simulink model "Bilateral_Ankle_Exo"  (R2017b)
settings: Solver=ode1  StartTime=0.0  StopTime=Inf  FixedStep=0.0002  RelTol=1e-3
PostLoadFcn:
  | , if any(exist('dsrtsu_mdlpostloadfcn', 'file') == [2, 3, 6]), try dsrtsu_mdlpostloadfcn('Execute', bdroot); catch fprintf('Error in PostLoadFcn (dsrtsu_mdlpostloadfcn) for model "%s":\n %s\n', bdroot, lasterr); end, end,
libraries: dsparch4 x12, rti1202lib_dio_class1 x8, rti1202lib_adc_class1 x8, rtican x5, rtiemclib x4, rti1202lib_dac_class1 x2, dsextras x1, rti1202lib_base x1, rtitasklib x1
(part 4 of 4)

== system Bilateral_Ankle_Exo/Sensor Data/IMU module/IMU/Subsystem6 ==
  Accel : Inport
  Data Type Conversion : DataTypeConversion  OutDataTypeStr=double
  Gain : Gain  Gain=4/32767
  Out1 : Outport
  wires:
  Data Type Conversion/1 -> Gain/1
  Gain/1 -> Out1/1
  Accel/1 -> Data Type Conversion/1

== system Bilateral_Ankle_Exo/Sensor Data/IMU module/IMU/Subsystem7 ==
  Accel : Inport
  Data Type Conversion : DataTypeConversion  OutDataTypeStr=double
  Gain : Gain  Gain=4/32767
  Out1 : Outport
  wires:
  Data Type Conversion/1 -> Gain/1
  Gain/1 -> Out1/1
  Accel/1 -> Data Type Conversion/1

== system Bilateral_Ankle_Exo/Sensor Data/IMU module/IMU/Subsystem8 ==
  Accel : Inport
  Data Type Conversion : DataTypeConversion  OutDataTypeStr=double
  Gain : Gain  Gain=4/32767
  Out1 : Outport
  wires:
  Data Type Conversion/1 -> Gain/1
  Gain/1 -> Out1/1
  Accel/1 -> Data Type Conversion/1

== system Bilateral_Ankle_Exo/RTI Data/RTI Data Store/RTI Data Store/RTI Data Store/RTI Data Store ==

== matlab function Bilateral_Ankle_Exo/Sensor Data/Ankle Encoder/Calibration_R ==
  data: encoder input; angle output; BT_RESET_ANKLE_R parameter boolean; ParmReg_R data_store_memory
function angle = process(encoder, BT_RESET_ANKLE_R)
    global ParmReg_R;
    angle_zero = ParmReg_R(3);


    if BT_RESET_ANKLE_R == 1
        angle_zero = encoder;
        ParmReg_R(3) = angle_zero;
    end

    angle = encoder - angle_zero;
end

== matlab function Bilateral_Ankle_Exo/Sensor Data/Motor Encoder/Calibration_L ==
  data: encoder input; BT_RESET_MOTOR_L parameter boolean; angle output; ParmReg_L data_store_memory
function angle = process(encoder, BT_RESET_MOTOR_L)
    global ParmReg_L;
    angle_zero = ParmReg_L(2);

    if BT_RESET_MOTOR_L == 1
        angle_zero = encoder;
        ParmReg_L(2) = angle_zero;
    end

    angle = encoder - angle_zero;
    
end

== matlab function Bilateral_Ankle_Exo/Sensor Data/Ankle Encoder/Mux ==
  data: x1 input; x output; x2 input
function x = mux(x1,x2)

x = [x1 x2];

== matlab function Bilateral_Ankle_Exo/Sensor Data/Torque module/Calibration_R ==
  data: vol input; torque output; load_vol_gain parameter double; load_vol_offset parameter double; BT_RESET_TORQUE_R parameter boolean; ParmReg_R data_store_memory
function torque = process(vol, load_vol_gain, load_vol_offset, BT_RESET_TORQUE_R)
%% 功能：电压-力矩转换与力矩归零
    global ParmReg_R;
    torque_zero = ParmReg_R(1);

    %%% 力矩归零
    if BT_RESET_TORQUE_R == 1
        torque_zero = vol*load_vol_gain + load_vol_offset;
        ParmReg_R(1) = torque_zero;
    end

    torque = vol*load_vol_gain + load_vol_offset - torque_zero;

end

== matlab function Bilateral_Ankle_Exo/Sensor Data/Motor Encoder/Mux1 ==
  data: x1 input; x output; x2 input; x3 input
function x = mux(x1,x2,x3)

x = [x1 x2 x3];

== matlab function Bilateral_Ankle_Exo/Sensor Data/FootSwitch module/Filter_R ==
  data: signal input; state output
function state = filter(signal)

%% 对足底开关信号进行滤波
% 滤波原则：上升沿无滤波，下降沿消抖滤波

Ts = 0.0002;
persistent foot_state;
persistent filter_time;

if isempty(foot_state)
    foot_state = 0;
    filter_time = 0;
end

if foot_state == 0
    if signal == 1
        foot_state = 1;
    else
        foot_state = 0;
    end
else
    if signal == 1
        foot_state = 1;
    else
        filter_time = filter_time + Ts;
        if filter_time > 0.1
            filter_time = 0;
            foot_state = 0;
        end
    end
end

state = foot_state;

end

== matlab function Bilateral_Ankle_Exo/Parameter Module/Control Parameter/Mux1 ==
  data: x1 input; x output; x2 input; x3 input; x4 input; x5 input; x6 input; reset input
function x = mux(x1,x2,x3,x4,x5,x6, reset)

if reset == 1
    x = [0 0 0 0 0 0];
else
    x = [x1 x2 x3 x4 x5 x6];
end

== matlab function Bilateral_Ankle_Exo/Parameter Module/Torque Parameter/Mux1 ==
  data: x1 input; x output; x2 input; x3 input; x4 input
function x = mux(x1,x2,x3,x4)

x = [x1 x2 x3,x4];

== matlab function Bilateral_Ankle_Exo/State_Module_r/State Machine ==
  data: mode_r output; footswitch_r input; state_r output; BT_RUN_R parameter boolean; BT_SLACK_R parameter boolean; BT_IDLE_R parameter boolean; BT_ERROR_R parameter boolean; stride_time_r output; BT_CALIB_R parameter boolean; stride_timer_r output
function [mode_r,state_r,stride_time_r,stride_timer_r] = StateMechine(footswitch_r, BT_RUN_R, BT_SLACK_R, BT_IDLE_R, BT_ERROR_R, BT_CALIB_R)

%% 定义寄存变量
persistent reg_stride_time;
persistent reg_stride_time_count;
persistent reg_mode;
persistent reg_state;
persistent bt_run;
persistent reg_last_switch;

if isempty(reg_stride_time)
    reg_stride_time = 1;
    reg_stride_time_count = 0;
    reg_mode = 1;
    reg_state = 1;
    bt_run = 0;
    reg_last_switch = 1;
end

%% 参数定义
Ts = 0.0002;
PP_StandSwing = 0.65;
max_stride_time = 1.5;
min_sride_time = 0.5;

%% 模式说明
IDLE_MODE  = 1;
WALK_MODE   = 2;
SLACK_MODE = 3;
CALIB_MODE = 4;
ERROR_MODE = 0;

%% 模式转换
if BT_RUN_R == 1
    bt_run = 1;
end
if BT_CALIB_R == 1
    reg_mode = CALIB_MODE;
end
if BT_SLACK_R == 1
    reg_mode = SLACK_MODE;
end
if BT_IDLE_R == 1
    reg_mode = IDLE_MODE;
end
if BT_ERROR_R == 1
    reg_mode = ERROR_MODE;
end
% 运行模式在swing->stance时切换
if bt_run == 1 && reg_last_switch == 0 && footswitch_r == 1
    reg_mode = WALK_MODE;
    bt_run = 0;
end
        
if reg_mode == WALK_MODE || reg_mode == IDLE_MODE
    if reg_last_switch == 0 && footswitch_r == 1
        reg_state = 1;
        
        if reg_stride_time_count < max_stride_time && reg_stride_time_count > min_sride_time
            reg_stride_time = 0.618*reg_stride_time + 0.382*reg_stride_time_count;
        end
        
        reg_stride_time_count = 0;
        
    elseif reg_state ==1 && reg_stride_time_count > PP_StandSwing * reg_stride_time
        reg_state = 0;
        reg_stride_time_count = reg_stride_time_count + Ts;
    else
        reg_stride_time_count = reg_stride_time_count + Ts;
    end
end

reg_last_switch = footswitch_r;
if reg_stride_time > max_stride_time
    reg_stride_time = max_stride_time;
elseif reg_stride_time < min_sride_time
    reg_stride_time = min_sride_time;
end

mode_r = reg_mode;
state_r = reg_state;
stride_time_r = reg_stride_time;
stride_timer_r = reg_stride_time_count;

end

== matlab function Bilateral_Ankle_Exo/State_Module_r/Mux1 ==
  data: x1 input; x output; x2 input; x3 input; x4 input
function x = mux(x1,x2,x3,x4)

x = [x1 x2 x3,x4];

== matlab function Bilateral_Ankle_Exo/Control Module/Controller_R ==
  data: state input; motor_vel_cmd_r output; torque input; ankle input; motor input; control_parm input; torque_trace_des input; torque_delta_trace_des input; lrn_cmd input; MODE_R parameter int8; FOLLOW_SLACK_ANGLE_R parameter double; TorqueMem_R data_store_memory; SWING_MAX_ANGLE_R parameter double; ParmReg_R data_store_memory
function motor_vel_cmd_r  = control(state,torque,ankle,motor,control_parm,torque_trace_des,torque_delta_trace_des,lrn_cmd, MODE_R,FOLLOW_SLACK_ANGLE_R,SWING_MAX_ANGLE_R)

global ParmReg_R;

%% 寄存变量声明
persistent calib_state;
persistent smooth_filter;
if isempty(calib_state)
    calib_state = 0;
    smooth_filter = 0;
end

%% 模式定义
IDLE_MODE  = 1;
WALK_MODE   = 2;
SLACK_MODE = 3;
CALIB_MODE = 4;
ERROR_MODE = 0;

%% 控制模式定义
FOLLOW_MODE = 1;
TORQUE_MODE = 2;

%% 参数定义
GearRatio = 5;
RadiusRatio = 40/108;
MotorTimeConstance = 0.05;
CALIB_SPEED = 30;
SLACK_SPEED = 30;
CALIB_TORQUE = 5;
CALIB_SLACK_ANGLE = 20;

%% 数据提取
STATE = state(1);
footstate = state(2);
stride_time = state(3);
stride_timer = state(4);

ankle_angle = ankle(1);
ankle_gyro = ankle(2);
motor_angle = motor(1);
motor_gyro = motor(2);

torque_measure = torque(1);
torque_delta = torque(2);
torque_des = torque_trace_des;
torque_delta_des = torque_delta_trace_des;

Kp = control_parm(1);
Kd = control_parm(2);
Ksp = control_parm(4);
Ksd = control_parm(5);
Ko = control_parm(6);
Ks = 2;

switch STATE
    case IDLE_MODE
        motor_vel_cmd_r = 0;
        calib_state = 0;
        
    case SLACK_MODE
        motor_vel_cmd_r = -SLACK_SPEED*GearRatio;
        
    case CALIB_MODE
        if calib_state == 0 && torque_measure < CALIB_TORQUE
            motor_vel_cmd_r = CALIB_SPEED*GearRatio;
        elseif calib_state == 0 && torque_measure > CALIB_TORQUE
            calib_state = 1;
            motor_vel_cmd_r = 0;
            motor_angle_zero = ParmReg_R(2) + motor_angle - CALIB_SLACK_ANGLE;
            ParmReg_R(2) = motor_angle_zero;
        else
            motor_vel_cmd_r = 0;
        end
        
    case WALK_MODE
        switch MODE_R
            
            case FOLLOW_MODE
                angle_error = ankle_angle - FOLLOW_SLACK_ANGLE_R - motor_angle*RadiusRatio;
                gyro_error = ankle_gyro*RadiusRatio;
                motor_vel_cmd_r = (Ksp*angle_error  + Ksd*gyro_error)*GearRatio/MotorTimeConstance;
                
            case TORQUE_MODE
                if footstate == 1
                    torque_error = torque_des - torque_measure;
                    torque_delta_error = torque_delta_des - torque_delta;
                    speed_des = Ko*torque_delta_des;
                    
                    angle_error = ankle_angle - FOLLOW_SLACK_ANGLE_R - motor_angle*RadiusRatio;
                    gyro_error = ankle_gyro*RadiusRatio;
                    motor_vel_cmd_r = (Ksp*angle_error  + Ksd*gyro_error)*GearRatio/MotorTimeConstance;
                    
                    if torque_des < 0.001
                        smooth_filter = smooth_filter + 0.05;
                        if smooth_filter > 1
                            smooth_filter = 1;
                        end
                    else
                        smooth_filter = 0;
                    end
                    
                    motor_vel_cmd_r = ((1-smooth_filter)*(Kp*torque_error + Kd*torque_delta_error + lrn_cmd + speed_des) + smooth_filter*(Ksp*angle_error  + Ksd*gyro_error)) * GearRatio / MotorTimeConstance;
                else
%                     angle_error = 0 - motor_angle*RadiusRatio;
%                     motor_vel_cmd = ( Ks * angle_error ) * GearRatio / MotorTimeConstance;
                    smooth_filter = 0;
                    angle_error = ankle_angle - FOLLOW_SLACK_ANGLE_R - motor_angle*RadiusRatio;
                    gyro_error = ankle_gyro*RadiusRatio;
                    motor_vel_cmd_r = (Ksp*angle_error  + Ksd*gyro_error)*GearRatio/MotorTimeConstance;
                end
            otherwise
                motor_vel_cmd_r = 0;
        end
        
    case ERROR_MODE
        motor_vel_cmd_r = 0;
        
    otherwise
        motor_vel_cmd_r = 0;
end


end

== matlab function Bilateral_Ankle_Exo/Control Module/Motor_R/MATLAB Function ==
  data: torque input; vel output; ankle input; motor input; motor_vel_cmd input; MAX_TORQUE parameter double; MAX_MOTOR_ANGLE parameter double; MIN_MOTOR_ANGLE parameter double; MAX_SPEED parameter double
function vel = fcn(torque,ankle,motor,motor_vel_cmd,MAX_TORQUE, MAX_MOTOR_ANGLE, MIN_MOTOR_ANGLE, MAX_SPEED)

motor_angle = motor(1);
torque_measure = torque(1);

if torque_measure > MAX_TORQUE
    vel = 0;
elseif motor_angle > MAX_MOTOR_ANGLE
    vel = 0;
elseif motor_angle < MIN_MOTOR_ANGLE
    vel = 0;
elseif motor_vel_cmd > MAX_SPEED
    vel = MAX_SPEED;
elseif motor_vel_cmd < - MAX_SPEED
    vel = - MAX_SPEED;
else
    vel = motor_vel_cmd;
end

end

== matlab function Bilateral_Ankle_Exo/Control Module/Torque Track R ==
  data: torque_parm_r input; torque_r input; torque_des_r output; torque_delta_des_r output; state_r input; TorqueMem_R data_store_memory; torque_trace_r output; torque_delta_trace_r output; torque_offset_r input; torque_error_r output
function [torque_des_r,torque_delta_des_r,torque_trace_r,torque_delta_trace_r,torque_error_r] = TorqueTrack(torque_parm_r,torque_r,state_r, torque_offset_r)

%% 寄存变量声明
global TorqueMem_R;

persistent last_footstate;
if isempty(last_footstate)
    last_footstate = 0;
end

%% 参数定义
Fs = 500;

%% 模式定义
IDLE_MODE  = 1;
WALK_MODE   = 2;

%% 数据提取
mode = state_r(1);
footstate = state_r(2);
stride_time = state_r(3);
stride_timer = state_r(4);

peak_torque = torque_parm_r(1);
rise_time = torque_parm_r(2);
peak_time = torque_parm_r(3);
fall_time = torque_parm_r(4);

torque_measure = torque_r(1);
troque_delta = torque_r(2);
stride_index = stride_timer*Fs + 1;
if stride_index > 750
    stride_index = 750;
end

%% 更新期望力矩曲线
if last_footstate == 0 && footstate == 1 && (mode == WALK_MODE || mode == IDLE_MODE)
    
    torque_track = zeros(1,750);
    
    torque_delta_track = zeros(1,750);
    time_index = 1:750;
    one_line = ones(1,750);
    index_peak = floor(peak_time/100*stride_time*Fs);
    index_rise = index_peak - floor(rise_time/100*stride_time*Fs);
    index_fall = index_peak + floor(fall_time/100*stride_time*Fs);
    
    %rise time前预拉紧阶段  ->使用向量代替循环以提高效率
    torque_track(1:floor(index_rise-1)) = time_index(1:floor(index_rise-1))/index_rise * torque_offset_r;
    
    % 上升阶段
    % 构造三次样条函数方程组
    A1 = [1,index_rise,index_rise^2,index_rise^3;
          1,index_peak,index_peak^2,index_peak^3;
          0,1,2*index_rise,3*index_rise^2;
          0,1,2*index_peak,3*index_peak^2];
    b1 = [torque_offset_r;peak_torque;0;0];
    parm1 = (A1\b1)';
    torque_track(floor(index_rise):floor(index_peak-1)) = parm1*[one_line(1:floor(index_peak-index_rise));time_index(floor(index_rise):floor(index_peak-1));time_index(floor(index_rise):floor(index_peak-1)).^2;time_index(floor(index_rise):floor(index_peak-1)).^3];
    torque_delta_track(index_rise:index_peak-1) = parm1(2:4)*[one_line(1:index_peak-index_rise);2*time_index(index_rise:index_peak-1);3*time_index(index_rise:index_peak-1).^2]*Fs;
    
    % 下降阶段
    A2 = [1,index_peak,index_peak^2,index_peak^3;
          1,index_fall,index_fall^2,index_fall^3;
          0,1,2*index_peak,3*index_peak^2;
          0,1,2*index_fall,3*index_fall^2];
    b2 = [peak_torque;0;0;0];
    parm2 = (A2\b2)';
    torque_track(floor(index_peak):floor(index_fall)) = parm2*[one_line(1:floor(index_fall+1-index_peak));time_index(floor(index_peak):floor(index_fall));time_index(floor(index_peak):floor(index_fall)).^2;time_index(floor(index_peak):floor(index_fall)).^3];
    
    %--------------------
    TorqueMem_R(1,1:750) = torque_track(1:750);
    %TorqueMem(2,1:750) = zeros(1,750);
    TorqueMem_R(3,1:750) = torque_delta_track(1:750);
    %TorqueMem(4,1:750) = zeros(1,750);
end

last_footstate = footstate;
TorqueMem_R(2,stride_index) = torque_measure;
TorqueMem_R(4,stride_index) = troque_delta;

if mode == WALK_MODE
    torque_des_r = TorqueMem_R(1,stride_index);
    torque_delta_des_r = TorqueMem_R(3,stride_index);
else
    torque_des_r = 0;
    torque_delta_des_r = 0;
end

torque_trace_r = TorqueMem_R(1:2,1:750);
torque_delta_trace_r = TorqueMem_R(3:4,1:750);

torque_error_r = torque_des_r - torque_r;

end

== matlab function Bilateral_Ankle_Exo/Control Module/LRN_R ==
  data: lrn_cmd_r output; state input; control_parm input; torque_parm input; BT_LRN_CLEAR_R parameter boolean; BT_LRN_ON_R parameter boolean; error_filter_k_r parameter double; time_delay_r parameter int32; lrn_mem_r output; TorqueMem_R data_store_memory; lrn_shrink_r parameter double
function [lrn_cmd_r, lrn_mem_r] = LRN_controller(state,control_parm,torque_parm, BT_LRN_CLEAR_R, BT_LRN_ON_R, error_filter_k_r, time_delay_r, lrn_shrink_r)

global TorqueMem_R;

persistent last_footstate;
persistent torque_error_memory;
persistent lrn_cmd_memory;
persistent last_torque_parm;

if isempty(last_footstate)
    last_footstate = 0;
    torque_error_memory = zeros(1,1000);
    lrn_cmd_memory = zeros(1,1000);
    last_torque_parm = [torque_parm(1) torque_parm(3)];
end

%% 参数定义
Fs = 500;

%% 模式定义
IDLE_MODE  = 1;
WALK_MODE   = 2;

%% 数据提取
mode = state(1);
footstate = state(2);
stride_time = state(3);
stride_timer = state(4);

Kl = control_parm(3);

stride_index = stride_timer*Fs + 1;
if stride_index > 750
    stride_index = 750;
end

if last_footstate == 0 && footstate == 1 && mode == WALK_MODE && BT_LRN_ON_R == 1
    error = TorqueMem_R(1,1:750) - TorqueMem_R(2,1:750);
    torque_error_memory(1:750) = (1-error_filter_k_r)*torque_error_memory(1:750) + error_filter_k_r*error;
    lrn_cmd_memory(1:750) = lrn_shrink_r*lrn_cmd_memory(1:750) + Kl*torque_error_memory(1:750);
end
    
if BT_LRN_CLEAR_R == 1 || last_torque_parm(1) ~= torque_parm(1) || last_torque_parm(2) ~= torque_parm(3)
    torque_error_memory = zeros(1,1000);
    lrn_cmd_memory = zeros(1,1000);
end

if mode == WALK_MODE
    if stride_index >= 750 - floor(time_delay_r)
        lrn_cmd_r = 0;
    else
        lrn_cmd_r = lrn_cmd_memory(1,stride_index + floor(time_delay_r));
    end
else
    lrn_cmd_r = 0;
end

last_footstate = footstate;
last_torque_parm = [torque_parm(1) torque_parm(3)];
lrn_mem_r = lrn_cmd_memory(1:750);


end

== matlab function Bilateral_Ankle_Exo/Sensor Data/Torque module/Calibration_L ==
  data: vol input; load_vol_gain parameter double; load_vol_offset parameter double; torque output; ParmReg_L data_store_memory; BT_RESET_TORQUE_L parameter boolean
function torque = process(vol, load_vol_gain, load_vol_offset, BT_RESET_TORQUE_L)
%% 功能：电压-力矩转换与力矩归零
    global ParmReg_L;
    torque_zero = ParmReg_L(1);

    %%% 力矩归零
    if BT_RESET_TORQUE_L == 1
        torque_zero = vol*load_vol_gain + load_vol_offset;
        ParmReg_L(1) = torque_zero;
    end

    torque = vol*load_vol_gain + load_vol_offset - torque_zero;

end

== matlab function Bilateral_Ankle_Exo/Sensor Data/Torque module/Mux_R ==
  data: x1 input; x output; x2 input
function x = mux(x1,x2)

x = [x1 x2];

== matlab function Bilateral_Ankle_Exo/Sensor Data/Ankle Encoder/Calibration_L ==
  data: encoder input; angle output; BT_RESET_ANKLE_L parameter boolean; ParmReg_L data_store_memory
function angle = process(encoder, BT_RESET_ANKLE_L)
    global ParmReg_L;
    angle_zero = ParmReg_L(3);

    if BT_RESET_ANKLE_L == 1
        angle_zero = encoder;
        ParmReg_L(3) = angle_zero;
    end

    angle = encoder - angle_zero;
end

== matlab function Bilateral_Ankle_Exo/Sensor Data/Torque module/MATLAB Function ==
  data: torque input; torque_dot output
function torque_dot = fcn(torque)

persistent data;
if isempty(data)
    data = ones(15,1);
end

data = [data(2:15);torque];

a1 = ones(15,1);
a2 = (1:15)';
A = [a1 a2];
x = A\data;

torque_dot = x(2)*5000;

== matlab function Bilateral_Ankle_Exo/Sensor Data/Torque module/Mux_L ==
  data: x1 input; x output; x2 input
function x = mux(x1,x2)

x = [x1 x2];

== matlab function Bilateral_Ankle_Exo/Sensor Data/EMG module/Preprocessing/MVC ==
  data: u input; y output; r_SOL_MIN parameter; r_SOL_MAX parameter
function y = fcn(u, r_SOL_MIN, r_SOL_MAX)

y = (u-r_SOL_MIN)/(r_SOL_MAX-r_SOL_MIN)

== matlab function Bilateral_Ankle_Exo/Sensor Data/EMG module/Preprocessing1/MVC ==
  data: u input; y output; r_M_GAS_MIN parameter; r_M_GAS_MAX parameter
function y = fcn(u, r_M_GAS_MIN, r_M_GAS_MAX)

y = (u-r_M_GAS_MIN)/(r_M_GAS_MAX-r_M_GAS_MIN)

== matlab function Bilateral_Ankle_Exo/Sensor Data/EMG module/Mux1 ==
  data: x1 input; x output; x2 input; x3 input; x4 input; x5 input; x6 input
function x = mux(x1,x2,x3,x4,x5,x6)

x = [x1 x2 x3 x4 x5 x6];

== matlab function Bilateral_Ankle_Exo/Sensor Data/EMG module/Preprocessing2/MVC ==
  data: u input; y output; r_L_GAS_MIN parameter; r_L_GAS_MAX parameter
function y = fcn(u, r_L_GAS_MIN, r_L_GAS_MAX)

y = (u-r_L_GAS_MIN)/(r_L_GAS_MAX-r_L_GAS_MIN)

== matlab function Bilateral_Ankle_Exo/Sensor Data/EMG module/Preprocessing3/MVC ==
  data: u input; y output; l_M_GAS_MIN parameter; l_M_GAS_MAX parameter
function y = fcn(u, l_M_GAS_MIN, l_M_GAS_MAX)

y = (u-l_M_GAS_MIN)/(l_M_GAS_MAX-l_M_GAS_MIN)

== matlab function Bilateral_Ankle_Exo/Sensor Data/EMG module/Preprocessing9/MVC ==
  data: u input; y output; l_L_GAS_MIN parameter; l_L_GAS_MAX parameter
function y = fcn(u, l_L_GAS_MIN, l_L_GAS_MAX)

y = (u-l_L_GAS_MIN)/(l_L_GAS_MAX-l_L_GAS_MIN)

== matlab function Bilateral_Ankle_Exo/Sensor Data/Ankle Encoder/Mux1 ==
  data: x1 input; x output; x2 input
function x = mux(x1,x2)

x = [x1 x2];

== matlab function Bilateral_Ankle_Exo/Sensor Data/Motor Encoder/Calibration_R ==
  data: encoder input; BT_RESET_MOTOR_R parameter boolean; angle output; ParmReg_R data_store_memory
function angle = process(encoder, BT_RESET_MOTOR_R)
    global ParmReg_R;
    angle_zero = ParmReg_R(2);

    if BT_RESET_MOTOR_R == 1
        angle_zero = encoder;
        ParmReg_R(2) = angle_zero;
    end

    angle = encoder - angle_zero;
    
end

== matlab function Bilateral_Ankle_Exo/Sensor Data/Motor Encoder/Mux3 ==
  data: x1 input; x output; x2 input; x3 input
function x = mux(x1,x2,x3)

x = [x1 x2 x3];

== matlab function Bilateral_Ankle_Exo/Sensor Data/FootSwitch module/Filter_L ==
  data: signal input; state output
function state = filter(signal)

%% 对足底开关信号进行滤波
% 滤波原则：上升沿无滤波，下降沿消抖滤波

Ts = 0.0002;
persistent foot_state;
persistent filter_time;

if isempty(foot_state)
    foot_state = 0;
    filter_time = 0;
end

if foot_state == 0
    if signal == 1
        foot_state = 1;
    else
        foot_state = 0;
    end
else
    if signal == 1
        foot_state = 1;
    else
        filter_time = filter_time + Ts;
        if filter_time > 0.1
            filter_time = 0;
            foot_state = 0;
        end
    end
end

state = foot_state;

end

== matlab function Bilateral_Ankle_Exo/State_Module_l/Mux1 ==
  data: x1 input; x output; x2 input; x3 input; x4 input
function x = mux(x1,x2,x3,x4)

x = [x1 x2 x3,x4];

== matlab function Bilateral_Ankle_Exo/State_Module_l/State Machine ==
  data: mode_l output; footswitch_l input; state_l output; BT_RUN_L parameter boolean; BT_SLACK_L parameter boolean; BT_IDLE_L parameter boolean; BT_ERROR_L parameter boolean; stride_time_l output; BT_CALIB_L parameter boolean; stride_timer_l output
function [mode_l,state_l,stride_time_l,stride_timer_l] = StateMechine(footswitch_l, BT_RUN_L, BT_SLACK_L, BT_IDLE_L, BT_ERROR_L, BT_CALIB_L)

%% 定义寄存变量
persistent reg_stride_time;
persistent reg_stride_time_count;
persistent reg_mode;
persistent reg_state;
persistent bt_run;
persistent reg_last_switch;

if isempty(reg_stride_time)
    reg_stride_time = 1;
    reg_stride_time_count = 0;
    reg_mode = 1;
    reg_state = 1;
    bt_run = 0;
    reg_last_switch = 1;
end

%% 参数定义
Ts = 0.0002;
PP_StandSwing = 0.65;
max_stride_time = 1.5;
min_sride_time = 0.5;

%% 模式说明
IDLE_MODE  = 1;
WALK_MODE   = 2;
SLACK_MODE = 3;
CALIB_MODE = 4;
ERROR_MODE = 0;

%% 模式转换
if BT_RUN_L == 1
    bt_run = 1;
end
if BT_CALIB_L == 1
    reg_mode = CALIB_MODE;
end
if BT_SLACK_L == 1
    reg_mode = SLACK_MODE;
end
if BT_IDLE_L == 1
    reg_mode = IDLE_MODE;
end
if BT_ERROR_L == 1
    reg_mode = ERROR_MODE;
end
% 运行模式在swing->stance时切换
if bt_run == 1 && reg_last_switch == 0 && footswitch_l == 1
    reg_mode = WALK_MODE;
    bt_run = 0;
end
        
if reg_mode == WALK_MODE || reg_mode == IDLE_MODE
    if reg_last_switch == 0 && footswitch_l == 1
        reg_state = 1;
        
        if reg_stride_time_count < max_stride_time && reg_stride_time_count > min_sride_time
            reg_stride_time = 0.618*reg_stride_time + 0.382*reg_stride_time_count;
        end
        
        reg_stride_time_count = 0;
        
    elseif reg_state ==1 && reg_stride_time_count > PP_StandSwing * reg_stride_time
        reg_state = 0;
        reg_stride_time_count = reg_stride_time_count + Ts;
    else
        reg_stride_time_count = reg_stride_time_count + Ts;
    end
end

reg_last_switch = footswitch_l;
if reg_stride_time > max_stride_time
    reg_stride_time = max_stride_time;
elseif reg_stride_time < min_sride_time
    reg_stride_time = min_sride_time;
end

mode_l = reg_mode;
state_l = reg_state;
stride_time_l = reg_stride_time;
stride_timer_l = reg_stride_time_count;

end

== matlab function Bilateral_Ankle_Exo/Control Module/Torque Track L ==
  data: torque_offset_l input; torque_parm_l input; torque_l input; state_l input; torque_des_l output; torque_delta_des_l output; TorqueMem_L data_store_memory; torque_trace_l output; torque_delta_trace_l output; torque_error_l output
function [torque_des_l,torque_delta_des_l,torque_trace_l,torque_delta_trace_l,torque_error_l] = TorqueTrack(torque_offset_l, torque_parm_l,torque_l,state_l)

%% 寄存变量声明
global TorqueMem_L;

persistent last_footstate;
if isempty(last_footstate)
    last_footstate = 0;
end

%% 参数定义
Fs = 500;

%% 模式定义
IDLE_MODE  = 1;
WALK_MODE   = 2;

%% 数据提取
mode = state_l(1);
footstate = state_l(2);
stride_time = state_l(3);
stride_timer = state_l(4);

peak_torque = torque_parm_l(1);
rise_time = torque_parm_l(2);
peak_time = torque_parm_l(3);
fall_time = torque_parm_l(4);

torque_measure = torque_l(1);
troque_delta = torque_l(2);
stride_index = stride_timer*Fs + 1;
if stride_index > 750
    stride_index = 750;
end

%% 更新期望力矩曲线
if last_footstate == 0 && footstate == 1 && (mode == WALK_MODE || mode == IDLE_MODE)
    
    torque_track = zeros(1,750);
    
    torque_delta_track = zeros(1,750);
    time_index = 1:750;
    one_line = ones(1,750);
    index_peak = floor(peak_time/100*stride_time*Fs);
    index_rise = index_peak - floor(rise_time/100*stride_time*Fs);
    index_fall = index_peak + floor(fall_time/100*stride_time*Fs);
    
    %rise time前预拉紧阶段  ->使用向量代替循环以提高效率
    torque_track(1:floor(index_rise-1)) = time_index(1:floor(index_rise-1))/index_rise * torque_offset_l;
    
    % 上升阶段
    % 构造三次样条函数方程组
    A1 = [1,index_rise,index_rise^2,index_rise^3;
          1,index_peak,index_peak^2,index_peak^3;
          0,1,2*index_rise,3*index_rise^2;
          0,1,2*index_peak,3*index_peak^2];
    b1 = [torque_offset_l;peak_torque;0;0];
    parm1 = (A1\b1)';
    torque_track(floor(index_rise):floor(index_peak-1)) = parm1*[one_line(1:floor(index_peak-index_rise));time_index(floor(index_rise):floor(index_peak-1));time_index(floor(index_rise):floor(index_peak-1)).^2;time_index(floor(index_rise):floor(index_peak-1)).^3];
    torque_delta_track(index_rise:index_peak-1) = parm1(2:4)*[one_line(1:index_peak-index_rise);2*time_index(index_rise:index_peak-1);3*time_index(index_rise:index_peak-1).^2]*Fs;
    
    % 下降阶段
    A2 = [1,index_peak,index_peak^2,index_peak^3;
          1,index_fall,index_fall^2,index_fall^3;
          0,1,2*index_peak,3*index_peak^2;
          0,1,2*index_fall,3*index_fall^2];
    b2 = [peak_torque;0;0;0];
    parm2 = (A2\b2)';
    torque_track(floor(index_peak):floor(index_fall)) = parm2*[one_line(1:floor(index_fall+1-index_peak));time_index(floor(index_peak):floor(index_fall));time_index(floor(index_peak):floor(index_fall)).^2;time_index(floor(index_peak):floor(index_fall)).^3];
    
    %--------------------
    TorqueMem_L(1,1:750) = torque_track(1:750);
    %TorqueMem(2,1:750) = zeros(1,750);
    TorqueMem_L(3,1:750) = torque_delta_track(1:750);
    %TorqueMem(4,1:750) = zeros(1,750);
end

last_footstate = footstate;
TorqueMem_L(2,stride_index) = torque_measure;
TorqueMem_L(4,stride_index) = troque_delta;

if mode == WALK_MODE
    torque_des_l = TorqueMem_L(1,stride_index);
    torque_delta_des_l = TorqueMem_L(3,stride_index);
else
    torque_des_l = 0;
    torque_delta_des_l = 0;
end

torque_trace_l = TorqueMem_L(1:2,1:750);
torque_delta_trace_l = TorqueMem_L(3:4,1:750);
torque_error_l = torque_des_l - torque_l;

end

== matlab function Bilateral_Ankle_Exo/Control Module/LRN_L ==
  data: torque_parm input; control_parm input; lrn_cmd_l output; state input; BT_LRN_CLEAR_L parameter boolean; BT_LRN_ON_L parameter boolean; error_filter_k_l parameter double; time_delay_l parameter int32; lrn_mem_l output; TorqueMem_L data_store_memory; lrn_shrink_l parameter double
function [lrn_cmd_l, lrn_mem_l] = LRN_controller(torque_parm,control_parm,state, BT_LRN_CLEAR_L, BT_LRN_ON_L, error_filter_k_l, time_delay_l, lrn_shrink_l)

global TorqueMem_L;

persistent last_footstate;
persistent torque_error_memory;
persistent lrn_cmd_memory;
persistent last_torque_parm;

if isempty(last_footstate)
    last_footstate = 0;
    torque_error_memory = zeros(1,1000);
    lrn_cmd_memory = zeros(1,1000);
    last_torque_parm = [torque_parm(1) torque_parm(3)];
end

%% 参数定义
Fs = 500;

%% 模式定义
IDLE_MODE  = 1;
WALK_MODE   = 2;

%% 数据提取
mode = state(1);
footstate = state(2);
stride_time = state(3);
stride_timer = state(4);

Kl = control_parm(3);

stride_index = stride_timer*Fs + 1;
if stride_index > 750
    stride_index = 750;
end

if last_footstate == 0 && footstate == 1 && mode == WALK_MODE && BT_LRN_ON_L == 1
    error = TorqueMem_L(1,1:750) - TorqueMem_L(2,1:750);
    torque_error_memory(1:750) = (1-error_filter_k_l)*torque_error_memory(1:750) + error_filter_k_l*error;
    lrn_cmd_memory(1:750) = lrn_shrink_l*lrn_cmd_memory(1:750) + Kl*torque_error_memory(1:750);
end

if BT_LRN_CLEAR_L == 1 || last_torque_parm(1) ~= torque_parm(1) || last_torque_parm(2) ~= torque_parm(3)
    torque_error_memory = zeros(1,1000);
    lrn_cmd_memory = zeros(1,1000);
end

if mode == WALK_MODE
    if stride_index >= 750 - floor(time_delay_l)
        lrn_cmd_l = 0;
    else
        lrn_cmd_l = lrn_cmd_memory(1,stride_index + floor(time_delay_l));
    end
else
    lrn_cmd_l = 0;
end

last_footstate = footstate;
last_torque_parm = [torque_parm(1) torque_parm(3)];
lrn_mem_l = lrn_cmd_memory(1:750);


end

== matlab function Bilateral_Ankle_Exo/Control Module/Controller_L ==
  data: control_parm input; lrn_cmd input; torque_trace_des input; torque_delta_trace_des input; state input; motor_vel_cmd_l output; torque input; ankle input; motor input; MODE_L parameter int8; FOLLOW_SLACK_ANGLE_L parameter double; TorqueMem_L data_store_memory; SWING_MAX_ANGLE_L parameter double; ParmReg_L data_store_memory
function motor_vel_cmd_l  = control(control_parm, lrn_cmd, torque_trace_des,torque_delta_trace_des,state,torque,ankle,motor,MODE_L,FOLLOW_SLACK_ANGLE_L,SWING_MAX_ANGLE_L)

global ParmReg_L;

%% 寄存变量声明
persistent calib_state;
persistent smooth_filter;
if isempty(calib_state)
    calib_state = 0;
    smooth_filter = 0;
end

%% 模式定义
IDLE_MODE  = 1;
WALK_MODE   = 2;
SLACK_MODE = 3;
CALIB_MODE = 4;
ERROR_MODE = 0;

%% 控制模式定义
FOLLOW_MODE = 1;
TORQUE_MODE = 2;

%% 参数定义
GearRatio = 5;
RadiusRatio = 40/108;
MotorTimeConstance = 0.05;
CALIB_SPEED = 30;
SLACK_SPEED = 30;
CALIB_TORQUE = 5;
CALIB_SLACK_ANGLE = 20;

%% 数据提取
STATE = state(1);
footstate = state(2);
stride_time = state(3);
stride_timer = state(4);

ankle_angle = ankle(1);
ankle_gyro = ankle(2);
motor_angle = motor(1);
motor_gyro = motor(2);

torque_measure = torque(1);
torque_delta = torque(2);
torque_des = torque_trace_des;
torque_delta_des = torque_delta_trace_des;

Kp = control_parm(1);
Kd = control_parm(2);
Ksp = control_parm(4);
Ksd = control_parm(5);
Ko = control_parm(6);
Ks = 2;

switch STATE
    case IDLE_MODE
        motor_vel_cmd_l = 0;
        calib_state = 0;
        
    case SLACK_MODE
        motor_vel_cmd_l = -SLACK_SPEED*GearRatio;
        
    case CALIB_MODE
        if calib_state == 0 && torque_measure < CALIB_TORQUE
            motor_vel_cmd_l = CALIB_SPEED*GearRatio;
        elseif calib_state == 0 && torque_measure > CALIB_TORQUE
            calib_state = 1;
            motor_vel_cmd_l = 0;
            motor_angle_zero = ParmReg_L(2) + motor_angle - CALIB_SLACK_ANGLE;
            ParmReg_L(2) = motor_angle_zero;
        else
            motor_vel_cmd_l = 0;
        end
        
    case WALK_MODE
        switch MODE_L
            
            case FOLLOW_MODE
                angle_error = ankle_angle - FOLLOW_SLACK_ANGLE_L - motor_angle*RadiusRatio;
                gyro_error = ankle_gyro*RadiusRatio;
                motor_vel_cmd_l = (Ksp*angle_error  + Ksd*gyro_error)*GearRatio/MotorTimeConstance;
                
            case TORQUE_MODE
                if footstate == 1
                    torque_error = torque_des - torque_measure;
                    torque_delta_error = torque_delta_des - torque_delta;
                    speed_des = Ko*torque_delta_des;
                    
                    angle_error = ankle_angle - FOLLOW_SLACK_ANGLE_L - motor_angle*RadiusRatio;
                    gyro_error = ankle_gyro*RadiusRatio;
                    motor_vel_cmd_l = (Ksp*angle_error  + Ksd*gyro_error)*GearRatio/MotorTimeConstance;
                    
                    if torque_des < 0.001
                        smooth_filter = smooth_filter + 0.05;
                        if smooth_filter > 1
                            smooth_filter = 1;
                        end
                    else
                        smooth_filter = 0;
                    end
                    
                    motor_vel_cmd_l = ((1-smooth_filter)*(Kp*torque_error + Kd*torque_delta_error + lrn_cmd + speed_des) + smooth_filter*(Ksp*angle_error  + Ksd*gyro_error)) * GearRatio / MotorTimeConstance;
                else
%                     angle_error = 0 - motor_angle*RadiusRatio;
%                     motor_vel_cmd = ( Ks * angle_error ) * GearRatio / MotorTimeConstance;
                    smooth_filter = 0;
                    angle_error = ankle_angle - FOLLOW_SLACK_ANGLE_L - motor_angle*RadiusRatio;
                    gyro_error = ankle_gyro*RadiusRatio;
                    motor_vel_cmd_l = (Ksp*angle_error  + Ksd*gyro_error)*GearRatio/MotorTimeConstance;
                end
            otherwise
                motor_vel_cmd_l = 0;
        end
        
    case ERROR_MODE
        motor_vel_cmd_l = 0;
        
    otherwise
        motor_vel_cmd_l = 0;
end


end

== matlab function Bilateral_Ankle_Exo/Control Module/Motor_L/MATLAB Function ==
  data: torque input; vel output; ankle input; motor input; motor_vel_cmd input; MAX_TORQUE parameter double; MAX_MOTOR_ANGLE parameter double; MIN_MOTOR_ANGLE parameter double; MAX_SPEED parameter double
function vel = fcn(torque,ankle,motor,motor_vel_cmd,MAX_TORQUE, MAX_MOTOR_ANGLE, MIN_MOTOR_ANGLE, MAX_SPEED)

motor_angle = motor(1);
torque_measure = torque(1);

if torque_measure > MAX_TORQUE
    vel = 0;
elseif motor_angle > MAX_MOTOR_ANGLE
    vel = 0;
elseif motor_angle < MIN_MOTOR_ANGLE
    vel = 0;
elseif motor_vel_cmd > MAX_SPEED
    vel = MAX_SPEED;
elseif motor_vel_cmd < - MAX_SPEED
    vel = - MAX_SPEED;
else
    vel = motor_vel_cmd;
end

end
